simulink library "Feeder3_lib"  (Simulink 8.1)
settings: Solver=ode45  StartTime=0.0  StopTime=10.0  RelTol=1e-3
values from neighbouring files (symbols this model uses):
  DER_REL = xlsread('DER_relay.xlsx')    [relay_settings_init.m]
  Ts = 100E-6    (= 0.0001)    [BANSHEE_init.m]    (also in Ghost_init.m)
undefined symbols (not defined in the file or in its folder): CBID, Left, type, V
libraries: cables_lib x12, breaker_lib x12, powerlib x7, transformer_lib x6, Load_lib x6, ssn_lib x3, PHIL_lib x2, rtio_generic_modbus x2, NREL_Diesel_Genset_lib x2, rtlab x2, powerlib_meascontrol x1, Motor_InductionMachine_lib x1
settings Model: Creator=re25624  LastModifiedBy=hptb1

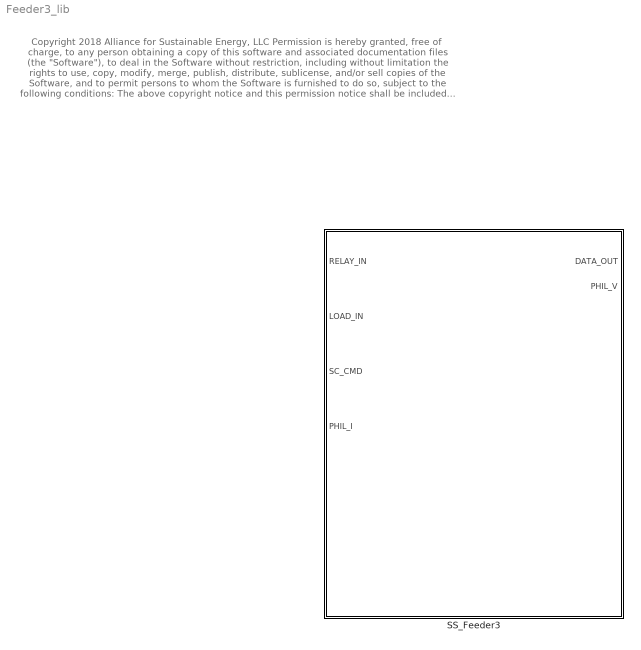
== system Feeder3_lib ==
  note: Copyright 2018 Alliance for Sustainable Energy, LLC
      |
      | Permission is hereby granted, free of charge, to any person obtaining a copy of this software
      | and associated documentation files (the "Software"), to deal in the Software without restriction,
      | including without limitation the rights to use, copy, modify, merge, publish, distribute, sublicense,
      | and/or sell copies of the Software, and to permit persons to whom the Software is furnished to do so,
      | subject to the following conditions:
      |
      | The above copyright notice and this permission notice shall be included in all copies or substantial portions of the Software.
      |
      | THE SOFTWARE IS PROVIDED "AS IS", WITHOUT WARRANTY OF ANY KIND, EXPRESS OR IMPLIED, INCLUDING
      | BUT NOT LIMITED TO THE WARRANTIES OF MERCHANTABILITY, FITNESS FOR A PARTICULAR PURPOSE AND
      | NONINFRINGEMENT. IN NO EVENT SHALL THE AUTHORS, THE COPYRIGHT HOLDERS, THE UNITED STATES,
      | THE UNITED STATES DEPARTMENT OF ENERGY, OR ANY OF THEIR EMPLOYEES BE LIABLE FOR ANY CLAIM,
      | DAMAGES OR OTHER LIABILITY, WHETHER IN AN ACTION OF CONTRACT, TORT OR OTHERWISE, ARISING FROM,
      | OUT OF OR IN CONNECTION WITH THE SOFTWARE OR THE USE OR OTHER DEALINGS IN THE SOFTWARE.
  SS_Feeder3 : Subsystem

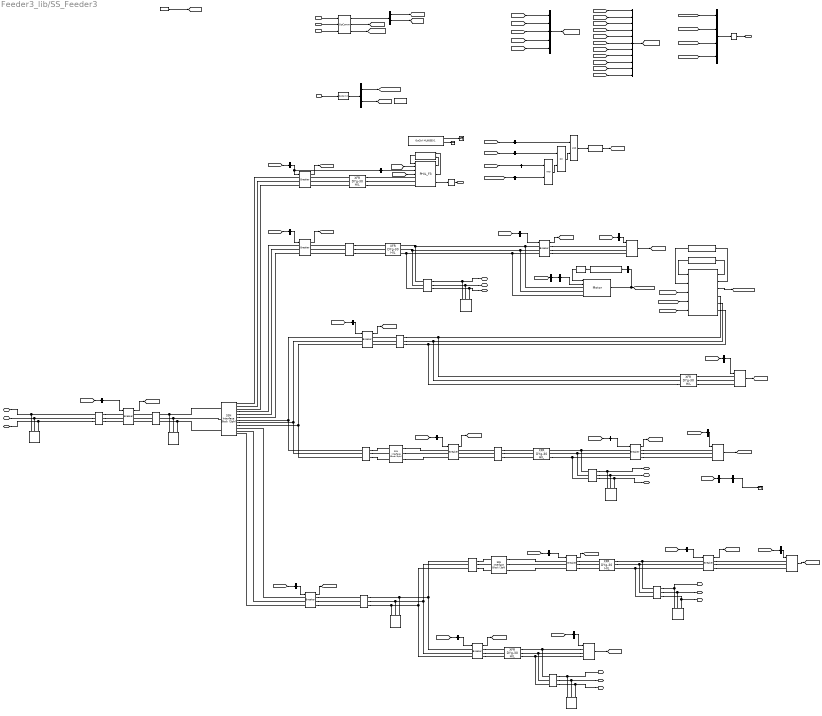
== system Feeder3_lib/SS_Feeder3 ==
  note: Copyright 2018 Alliance for Sustainable Energy, LLC
      |
      | Permission is hereby granted, free of charge, to any person obtaining a copy of this software
      | and associated documentation files (the "Software"), to deal in the Software without restriction,
      | including without limitation the rights to use, copy, modify, merge, publish, distribute, sublicense,
      | and/or sell copies of the Software, and to permit persons to whom the Software is furnished to do so,
      | subject to the following conditions:
      |
      | The above copyright notice and this permission notice shall be included in all copies or substantial portions of the Software.
      |
      | THE SOFTWARE IS PROVIDED "AS IS", WITHOUT WARRANTY OF ANY KIND, EXPRESS OR IMPLIED, INCLUDING
      | BUT NOT LIMITED TO THE WARRANTIES OF MERCHANTABILITY, FITNESS FOR A PARTICULAR PURPOSE AND
      | NONINFRINGEMENT. IN NO EVENT SHALL THE AUTHORS, THE COPYRIGHT HOLDERS, THE UNITED STATES,
      | THE UNITED STATES DEPARTMENT OF ENERGY, OR ANY OF THEIR EMPLOYEES BE LIABLE FOR ANY CLAIM,
      | DAMAGES OR OTHER LIABILITY, WHETHER IN AN ACTION OF CONTRACT, TORT OR OTHERWISE, ARISING FROM,
      | OUT OF OR IN CONNECTION WITH THE SOFTWARE OR THE USE OR OTHER DEALINGS IN THE SOFTWARE.
  note: PHIL interface
  note: connect to F1
  note: connect to F2
  note: connect to F2
  note: connect to F2
  note: Signal for this Cb will come from a SEL relay
  note: Logic to protect against situation where there is no voltage
      | source at F3 side of PHIL. If no voltage source is available current is not injected back to F3
  RELAY_IN : Inport
  LOAD_IN : Inport  Port=2
  SC_CMD : Inport  Port=3
  PHIL_I : Inport  Port=4
  1000 kVA : transformer_lib/XFR DYg-30 HIL  Rating=1000  Vp=13800  Vs=480  Z=5.56  XR=5.49
  1000 kVA1 : transformer_lib/XFR DYg-30 HIL  Rating=1000  Vp=13800  Vs=480  Z=5.56  XR=5.49
  200 HP chiller compressor : Load_lib/200 HP chiller compressor
  2000 kVA : transformer_lib/XFR DYg-30 HIL  Rating=2000  Vp=13800  Vs=480  Z=5.75  XR=5.7
  2000 kVA1 : transformer_lib/XFR DYg-30 HIL  Rating=2000  Vp=13800  Vs=480  Z=5.75  XR=5.7
  2500 kVA : transformer_lib/XFR DYg-30 HIL  Rating=2500  Vp=13800  Vs=480  Z=5.75  XR=6.6
  2500 kVA1 : transformer_lib/XFR DYg-30 HIL  Rating=5000  Vp=13800  Vs=4160  Z=5.75  XR=6.6
  448 kvar inductor at 13.8kV  to cancel kvar produced by the stublines1 : powerlib/Elements/Three-Phase Parallel RLC Load  LConnTagsString=A|B|C  Configuration=Y (grounded)  NominalVoltage=13800  NominalFrequency=60  ActivePower=10e3  InductivePower=448e3  CapacitivePower=0  Measurements=None  LoadType=constant Z
  5 kvar inductor at 480V  to cancel kvar produced by the stublines : powerlib/Elements/Three-Phase Parallel RLC Load  LConnTagsString=A|B|C  Configuration=Y (grounded)  NominalVoltage=480  NominalFrequency=60  ActivePower=1e3  InductivePower=5e3  CapacitivePower=0  Measurements=None  LoadType=constant Z
  500kcmil-Mutual{1..2,4,9} (4 alike) : cables_lib/500kcmil-Mutual  length=10  par_sets=1  ratio=3
  500kcmil-Mutual3 : cables_lib/500kcmil-Mutual  length=100  par_sets=1  ratio=3
  500kcmil-Mutual5 : cables_lib/500kcmil-Mutual  length=1000  par_sets=1  ratio=3
  6 kvar inductor at 480V  to cancel kvar produced by the stublines1 : powerlib/Elements/Three-Phase Parallel RLC Load  LConnTagsString=A|B|C  Configuration=Y (grounded)  NominalVoltage=480  NominalFrequency=60  ActivePower=1e3  InductivePower=6e3  CapacitivePower=0  Measurements=None  LoadType=constant Z
  6 kvar inductor at 480V  to cancel kvar produced by the stublines2 : powerlib/Elements/Three-Phase Parallel RLC Load  LConnTagsString=A|B|C  Configuration=Y (grounded)  NominalVoltage=480  NominalFrequency=60  ActivePower=1e3  InductivePower=6e3  CapacitivePower=0  Measurements=None  LoadType=constant Z
  6 kvar inductor at 480V  to cancel kvar produced by the stublines3 : powerlib/Elements/Three-Phase Parallel RLC Load  LConnTagsString=A|B|C  Configuration=Y (grounded)  NominalVoltage=480  NominalFrequency=60  ActivePower=0  InductivePower=6e3  CapacitivePower=0  Measurements=None  LoadType=constant Z
  AIN_AOUT_ML605EX1 : PHIL_lib/AIN_AOUT_ML605EX1
  Bus Creator2 : BusCreator
  Bus Creator3 : BusCreator  Inputs=5
  Bus Creator5 : BusCreator  Inputs=11
  Bus Selector : BusSelector  OutputSignals=motor
  Bus Selector1 : BusSelector  OutputSignals=F3_CB_4
  Bus Selector10 : BusSelector  OutputSignals=F3_CB_5
  Bus Selector11 : BusSelector  OutputSignals=P6
  Bus Selector12 : BusSelector  OutputSignals=F3_CB_9
  Bus Selector13 : BusSelector  OutputSignals=F3_CB_3
  Bus Selector14 : BusSelector  OutputSignals=F3_CB_8
  Bus Selector15 : BusSelector  OutputSignals=CHP_cmds,IO_scaling
  Bus Selector17 : BusSelector  OutputSignals=RPM
  Bus Selector18 : BusSelector  OutputSignals=LoadProfile,TestSeq
  Bus Selector19 : BusSelector  OutputSignals=Logic_trip
  Bus Selector2 : BusSelector  OutputSignals=C6
  Bus Selector20 : BusSelector  OutputSignals=ena2
  Bus Selector21 : BusSelector  OutputSignals=F3_PCC
  Bus Selector22 : BusSelector  OutputSignals=F3_CB_10
  Bus Selector23 : BusSelector  OutputSignals=fault
  Bus Selector24 : BusSelector  OutputSignals=loc4
  Bus Selector25 : BusSelector  OutputSignals=Status
  Bus Selector26 : BusSelector  OutputSignals=Status
  Bus Selector27 : BusSelector  OutputSignals=Status
  Bus Selector28 : BusSelector  OutputSignals=cb.cb_meas.Status
  Bus Selector3 : BusSelector  OutputSignals=P4
  Bus Selector4 : BusSelector  OutputSignals=I6
  Bus Selector5 : BusSelector  OutputSignals=C5
  Bus Selector6 : BusSelector  OutputSignals=F3_CB_2
  Bus Selector7 : BusSelector  OutputSignals=F3_CB_7
  Bus Selector8 : BusSelector  OutputSignals=F3_CB_6
  Bus Selector9 : BusSelector  OutputSignals=F3_CB_1
  C1 : cables_lib/500kcmil-Mutual  length=10  par_sets=1  ratio=3
  C2 : cables_lib/500kcmil-Mutual  length=10  par_sets=1  ratio=3
  C301 : cables_lib/500kcmil-Mutual  length=2500  par_sets=1  ratio=3
  C302 : cables_lib/4//0AWG-Mutual  length=2000  par_sets=1  ratio=3
  C303 : cables_lib/500kcmil-Mutual  length=2000  par_sets=1  ratio=3
  C304 : cables_lib/4//0AWG-Mutual  length=1500  par_sets=2  ratio=3
  CHP_Modbus : rtio_generic_modbus/Modbus device  conf_name=CHP_modbus.opal  conf_name_mask=CHP_modbus.xls  sample_time=Ts
  Critical_5 : Load_lib/Dynamic_Load  V=480  kVA=1000  PF=0.9  Ts=Ts
  Critical_6 : Load_lib/Dynamic_Load  V=480  kVA=800  PF=0.9  Ts=Ts
  Data Type Conversion : DataTypeConversion  OutDataTypeStr=double
  F3_CB_{1..6,8..11} (10 alike) : breaker_lib/Breaker  Ts=Ts  mech_delay=cb_mech_delay
  F3_PCC : breaker_lib/Breaker  Ts=Ts  mech_delay=cb_mech_delay
  First-Order Filter : powerlib_meascontrol/Filters/First-Order Filter  FilterType=Lowpass  Tc=10e-3  Ts=Ts  Initialize=on  Vac_Init=[0, 0, 60]  Vdc_Init=0  PlotResponse=off  FreqRange="[0,  200,  1]"
  GEN2_Modbus : rtio_generic_modbus/Modbus device  conf_name=GEN2_modbus.opal  conf_name_mask=GEN2_modbus.xls  sample_time=Ts
  Goto Tag Visibility : GotoTagVisibility  GotoTag=phil_ctrl
  Interruptible_6 : Load_lib/Dynamic_Load  V=480  kVA=600  PF=0.9  Ts=Ts
  Logical Operator : Logic  AllPortsSameDT=off  OutDataTypeStr=boolean
  Logical Operator1 : Logic  Operator=OR  AllPortsSameDT=off  OutDataTypeStr=boolean
  Logical Operator2 : Logic  AllPortsSameDT=off  OutDataTypeStr=boolean
  Losses1 : powerlib/Elements/Three-Phase Parallel RLC Load  LConnTagsString=A|B|C  Configuration=Y (grounded)  NominalVoltage=13800  NominalFrequency=60  ActivePower=1e3  InductivePower=0  CapacitivePower=0  Measurements=None  LoadType=constant Z
  Losses4 : powerlib/Elements/Three-Phase Parallel RLC Load  LConnTagsString=A|B|C  Configuration=Y (grounded)  NominalVoltage=13800  NominalFrequency=60  ActivePower=1e3  InductivePower=0  CapacitivePower=0  Measurements=None  LoadType=constant Z
  Memory : Memory
  Memory1 : Memory
  Motor : Motor_InductionMachine_lib/Motor
  NGCHP_Generator : Subsystem
  OpComm1 : rtlab/OpComm  nbport=3  groupe_acq=1  subsys_rate=0  st=0  Synchronization=on  Interpolation=on  Threshold=1.0  Missed_Data=off  Sim_Time=off  Samples=off  dynSigOut=off  from_console=0  warning_done=off  writeOpCommFile=off  Offset=off
  OpComm2 : rtlab/OpComm  nbport=1  groupe_acq=1  subsys_rate=0  st=0  Synchronization=on  Interpolation=on  Threshold=1.0  Missed_Data=off  Sim_Time=off  Samples=off  dynSigOut=off  from_console=1  warning_done=off  writeOpCommFile=off  Offset=off
  OpCtrl ML605EX1 : rtio_opalrt_ml605ex1/OpCtrl ML605EX1  CtrlName='ML605EX1 Ctrl'  boardid=4  BitstreamFilename=ML605_2-EX-0029-2_2_4_33-32AIO_16DIO16SelectableDIO-10-01.bin  numconfig=-1  mode=Master  externalClock=off  decimRtsi=0  calibIO=off  SampleTime=0  loadinport=-1
  PHIL_F3 : PHIL_lib/PHIL_F3
  Priority_4 : Load_lib/Dynamic_Load  V=480  kVA=600  PF=0.9  Ts=Ts
  Priority_6 : Load_lib/Dynamic_Load  V=480  kVA=1000  PF=0.9  Ts=Ts
  SSN Interface Block (3ph)1 : ssn_lib/SSN Interface Block (3ph)  nb_phase=3  nb_port=2  p1_type=V-type(Left)  p2_type=V-type (Right)  p3_type=V-type(Left)  p4_type=V-type(Left)  p5_type=V-type(Left)  p6_type=V-type(Left)  p7_type=V-type(Left)  p8_type=V-type(Left)  p9_type=V-type(Left)  p10_type=V-type(Left)  p11_type=V-type(Left)  p12_type=V-type(Left)  p13_type=V-type(Left)  p14_type=V-type(Left)  p15_type=V-type(Left)  p16_type=V-type(Left)  I_port_shunt_resistance=1e9
  SSN Interface Block (3ph)2 : ssn_lib/SSN Interface Block (3ph)  nb_phase=3  nb_port=2  p1_type=V-type(Left)  p2_type=V-type (Right)  p3_type=V-type(Left)  p4_type=V-type(Left)  p5_type=V-type(Left)  p6_type=V-type(Left)  p7_type=V-type(Left)  p8_type=V-type(Left)  p9_type=V-type(Left)  p10_type=V-type(Left)  p11_type=V-type(Left)  p12_type=V-type(Left)  p13_type=V-type(Left)  p14_type=V-type(Left)  p15_type=V-type(Left)  p16_type=V-type(Left)  I_port_shunt_resistance=1e9
  SSN Interface Block (3ph)5 : ssn_lib/SSN Interface Block (3ph)  nb_phase=3  nb_port=5  p1_type=V-type(Left)  p2_type=V-type (Right)  p3_type=V-type (Right)  p4_type=V-type (Right)  p5_type=V-type (Right)  p6_type=V-type(Left)  p7_type=V-type(Left)  p8_type=V-type(Left)  p9_type=V-type(Left)  p10_type=V-type(Left)  p11_type=V-type(Left)  p12_type=V-type(Left)  p13_type=V-type(Left)  p14_type=V-type(Left)  p15_type=V-type(Left)  p16_type=V-type(Left)  I_port_shunt_resistance=1e9
  "State " : Constant  Value=0
  Terminator : Terminator
  Terminator1 : Terminator
  Terminator5 : Terminator
  A_CB_4 : PMIOPort  Port=1  Side=Right
  B_CB_4 : PMIOPort  Port=2  Side=Right
  C_CB_4 : PMIOPort  Port=3  Side=Right
  A_CB_5 : PMIOPort  Port=4  Side=Right
  B_CB_5 : PMIOPort  Port=5  Side=Right
  C_CB_5 : PMIOPort  Port=6  Side=Right
  A_CB_6 : PMIOPort  Port=7  Side=Right
  B_CB_6 : PMIOPort  Port=8  Side=Right
  C_CB_6 : PMIOPort  Port=9  Side=Right
  A_CB_7 : PMIOPort  Port=10  Side=Right
  B_CB_7 : PMIOPort  Port=11  Side=Right
  C_CB_7 : PMIOPort  Port=12  Side=Right
  PCC_A : PMIOPort  Port=13  Side=Left
  PCC_B : PMIOPort  Port=14  Side=Left
  PCC_C : PMIOPort  Port=15  Side=Left
  DATA_OUT : Outport
  PHIL_V : Outport  Port=2
  tag scope: phil_ctrl=scoped
  wires:
  PHIL_F3/2 -> AIN_AOUT_ML605EX1/1
  Data Type Conversion/1 -> [Vsrc_con]
  [Vsrc_con] -> PHIL_F3/4
  Logical Operator/1 -> Data Type Conversion/1
  Logical Operator1/1 -> Logical Operator/2
  Logical Operator2/1 -> Logical Operator1/2
  Bus Selector27/1 -> Logical Operator2/1  "<Status>"
  Bus Selector28/1 -> Logical Operator2/2  "<Status>"
  [NG_CHP_DATA] -> Bus Selector28/1
  Bus Selector26/1 -> Logical Operator1/1  "<Status>"
  [F3_PCC] -> Bus Selector26/1
  Bus Selector25/1 -> Logical Operator/1  "<Status>"
  [F3_CB_3] -> Bus Selector27/1  "F3_CB_3"
  [F3_CB_10] -> Bus Selector25/1
  Bus Selector24/1 -> Terminator5/1  "<loc4>"
  Bus Selector23/1 -> Bus Selector24/1  "<fault>"
  [TestSeq] -> Bus Selector23/1
  AIN_AOUT_ML605EX1/1 -> PHIL_F3/1
  PHIL_F3/1 -> AIN_AOUT_ML605EX1/2
  First-Order Filter/1 -> Motor/1
  [TestSeq] -> NGCHP_Generator/5(testseq)
  [MOTOR_DATA] -> Bus Creator2/4  "MOTOR_DATA"
  Motor/1 -> [MOTOR_DATA], Bus Selector17/1
  OpCtrl ML605EX1/2 -> Terminator1/1
  OpCtrl ML605EX1/1 -> Terminator/1
  Bus Selector15/2 -> [phil_ctrl]  "<IO_scaling>"
  Bus Selector20/1 -> Motor/2  "<ena2>"
  [PHIL_I] -> PHIL_F3/2
  Bus Selector19/1 -> PHIL_F3/3  "<Logic_trip>"
  PHIL_F3/3 -> Memory1/1
  Memory1/1 -> PHIL_V/1
  Bus Selector22/1 -> F3_CB_10/1, Bus Selector19/1  "<F3_CB_10>"
  F3_CB_10/1 -> [F3_CB_10]
  Bus Selector18/2 -> [TestSeq]  "<TestSeq>"
  Bus Selector18/1 -> [LOAD_IN]  "<LoadProfile>"
  PHIL_I/1 -> OpComm1/3
  OpComm1/3 -> [PHIL_I]
  [F3_CB_10] -> Bus Creator5/10  "F3_CB_10"
  [RELAY_IN] -> Bus Selector22/1
  Bus Selector15/1 -> [NGCHP_Gen]  "<CHP_cmds>"
  CHP_Modbus/1 -> NGCHP_Generator/2(ModbusIn1)
  NGCHP_Generator/2(ModbusOutCHP) -> CHP_Modbus/1
  [heat_load] -> NGCHP_Generator/4(Heat Load MBtu/hrs)
  NGCHP_Generator/3(Gen_meas) -> [NG_CHP_DATA]
  NGCHP_Generator/1(ModbusOut) -> GEN2_Modbus/1  "Gen_meas"
  GEN2_Modbus/1 -> NGCHP_Generator/1(ModbusIn)
  [NGCHP_Gen] -> NGCHP_Generator/3(console)
  [RELAY_IN] -> Bus Selector21/1
  Bus Selector21/1 -> F3_PCC/1  "<F3_PCC>"
  Bus Selector/1 -> Bus Selector20/1  "<motor>"
  [TestSeq] -> Bus Selector/1
  200 HP chiller compressor/1 -> First-Order Filter/1
  Bus Selector17/1 -> 200 HP chiller compressor/1  "<RPM>"
  [NG_CHP_DATA] -> Bus Creator2/3  "NG_CHP_DATA"
  [LOAD_DATA] -> Bus Creator2/2  "LOAD_DATA"
  [CB_DATA] -> Bus Creator2/1  "CB_DATA"
  Bus Creator2/1 -> Memory/1
  OpComm2/1 -> Bus Selector15/1
  "State "/1 -> [heat_load]  "Heat Load MBtu/hr"
  Memory/1 -> DATA_OUT/1
  SC_CMD/1 -> OpComm2/1
  [F3_CB_9] -> Bus Creator5/9  "F3_CB_9"
  [F3_CB_8] -> Bus Creator5/8  "F3_CB_8"
  [RELAY_IN] -> Bus Selector14/1
  Bus Selector14/1 -> F3_CB_8/1  "<F3_CB_8>"
  F3_CB_8/1 -> [F3_CB_8]
  [RELAY_IN] -> Bus Selector12/1
  Bus Selector12/1 -> F3_CB_9/1  "<F3_CB_9>"
  F3_CB_9/1 -> [F3_CB_9]
  [LOAD_P6] -> Bus Creator3/5  "F3_P6"
  Priority_6/1 -> [LOAD_P6]
  Bus Selector11/1 -> Priority_6/1  "<P6>"
  [LOAD_IN] -> Bus Selector11/1
  [F3_PCC] -> Bus Creator5/11  "F3_PCC"
  F3_PCC/1 -> [F3_PCC]
  F3_CB_11/1 -> [F3_CB_7]
  [RELAY_IN] -> Bus Selector13/1
  Bus Selector13/1 -> F3_CB_3/1  "<F3_CB_3>"
  [RELAY_IN] -> Bus Selector10/1
  Bus Selector10/1 -> F3_CB_5/1  "<F3_CB_5>"
  [RELAY_IN] -> Bus Selector9/1
  Bus Selector9/1 -> F3_CB_1/1  "<F3_CB_1>"
  [RELAY_IN] -> Bus Selector8/1
  Bus Selector8/1 -> F3_CB_6/1  "<F3_CB_6>"
  [RELAY_IN] -> Bus Selector7/1
  Bus Selector7/1 -> F3_CB_11/1  "<F3_CB_7>"
  [RELAY_IN] -> Bus Selector6/1
  Bus Selector6/1 -> F3_CB_2/1  "<F3_CB_2>"
  OpComm1/2 -> [RELAY_IN]
  RELAY_IN/1 -> OpComm1/2
  [RELAY_IN] -> Bus Selector1/1
  Bus Creator5/1 -> [CB_DATA]
  [F3_CB_4] -> Bus Creator5/4  "F3_CB_4"
  [F3_CB_2] -> Bus Creator5/2  "F3_CB_2"
  [F3_CB_3] -> Bus Creator5/3  "F3_CB_3"
  [F3_CB_6] -> Bus Creator5/6  "F3_CB_6"
  [F3_CB_7] -> Bus Creator5/7  "F3_CB_7"
  [F3_CB_5] -> Bus Creator5/5  "F3_CB_5"
  [F3_CB_1] -> Bus Creator5/1  "F3_CB_1"
  F3_CB_5/1 -> [F3_CB_5]
  F3_CB_1/1 -> [F3_CB_1]
  F3_CB_6/1 -> [F3_CB_6]
  F3_CB_2/1 -> [F3_CB_2]
  F3_CB_3/1 -> [F3_CB_3]
  F3_CB_4/1 -> [F3_CB_4]
  Bus Creator3/1 -> [LOAD_DATA]  "LOAD"
  [LOAD_P4] -> Bus Creator3/4  "F3_P4"
  [LOAD_I6] -> Bus Creator3/3  "F3_I6"
  [LOAD_C5] -> Bus Creator3/1  "F3_C5"
  [LOAD_C6] -> Bus Creator3/2  "F3_C6"
  Critical_5/1 -> [LOAD_C5]
  Interruptible_6/1 -> [LOAD_I6]
  Priority_4/1 -> [LOAD_P4]
  Critical_6/1 -> [LOAD_C6]
  Bus Selector5/1 -> Critical_5/1  "<C5>"
  Bus Selector4/1 -> Interruptible_6/1  "<I6>"
  Bus Selector3/1 -> Priority_4/1  "<P4>"
  Bus Selector2/1 -> Critical_6/1  "<C6>"
  [LOAD_IN] -> Bus Selector5/1
  [LOAD_IN] -> Bus Selector4/1
  [LOAD_IN] -> Bus Selector3/1
  [LOAD_IN] -> Bus Selector2/1
  OpComm1/1 -> Bus Selector18/1
  LOAD_IN/1 -> OpComm1/1
  Bus Selector1/1 -> F3_CB_4/1  "<F3_CB_4>"
  connections:
  F3_CB_11/RConn3 -- Priority_4/LConn3
  F3_CB_11/RConn1 -- Priority_4/LConn1
  2500 kVA1/RConn1 -- PHIL_F3/LConn1
  2500 kVA1/RConn2 -- PHIL_F3/LConn2
  2500 kVA1/RConn3 -- PHIL_F3/LConn3
  2500 kVA1/LConn3 -- F3_CB_10/RConn3
  2500 kVA1/LConn1 -- F3_CB_10/RConn1
  2500 kVA1/LConn2 -- F3_CB_10/RConn2
  F3_CB_10/LConn1 -- SSN Interface Block (3ph)5/RConn1
  F3_CB_10/LConn2 -- SSN Interface Block (3ph)5/RConn2
  F3_CB_10/LConn3 -- SSN Interface Block (3ph)5/RConn3
  F3_CB_1/RConn3 -- C301/LConn3
  F3_CB_1/RConn2 -- C301/LConn2
  F3_CB_1/RConn1 -- C301/LConn1
  SSN Interface Block (3ph)1/RConn3 -- F3_CB_6/LConn3
  SSN Interface Block (3ph)1/RConn2 -- F3_CB_6/LConn2
  SSN Interface Block (3ph)1/RConn1 -- F3_CB_6/LConn1
  F3_CB_1/LConn3 -- SSN Interface Block (3ph)5/RConn12
  F3_CB_1/LConn1 -- SSN Interface Block (3ph)5/RConn10
  F3_CB_1/LConn2 -- SSN Interface Block (3ph)5/RConn11
  C2/RConn3 -- SSN Interface Block (3ph)2/LConn3
  C2/RConn1 -- SSN Interface Block (3ph)2/LConn1
  C2/RConn2 -- SSN Interface Block (3ph)2/LConn2
  SSN Interface Block (3ph)2/RConn1 -- F3_CB_2/LConn1
  SSN Interface Block (3ph)2/RConn2 -- F3_CB_2/LConn2
  SSN Interface Block (3ph)2/RConn3 -- F3_CB_2/LConn3
  500kcmil-Mutual5/LConn3 -- 448 kvar inductor at 13.8kV  to cancel kvar produced by the stublines1/LConn3 -- PCC_C/RConn1
  500kcmil-Mutual5/LConn2 -- 448 kvar inductor at 13.8kV  to cancel kvar produced by the stublines1/LConn2 -- PCC_B/RConn1
  448 kvar inductor at 13.8kV  to cancel kvar produced by the stublines1/LConn1 -- 500kcmil-Mutual5/LConn1 -- PCC_A/RConn1
  Losses4/LConn3 -- SSN Interface Block (3ph)5/LConn3 -- 500kcmil-Mutual3/RConn3
  Losses4/LConn2 -- SSN Interface Block (3ph)5/LConn2 -- 500kcmil-Mutual3/RConn2
  Losses4/LConn1 -- SSN Interface Block (3ph)5/LConn1 -- 500kcmil-Mutual3/RConn1
  C1/RConn1 -- SSN Interface Block (3ph)1/LConn1
  C1/RConn3 -- SSN Interface Block (3ph)1/LConn3
  C1/RConn2 -- SSN Interface Block (3ph)1/LConn2
  F3_CB_11/LConn3 -- 1000 kVA/RConn3 -- 500kcmil-Mutual4/LConn3
  500kcmil-Mutual5/RConn3 -- F3_PCC/LConn3
  500kcmil-Mutual5/RConn2 -- F3_PCC/LConn2
  500kcmil-Mutual5/RConn1 -- F3_PCC/LConn1
  500kcmil-Mutual3/LConn2 -- F3_PCC/RConn2
  500kcmil-Mutual3/LConn1 -- F3_PCC/RConn1
  500kcmil-Mutual3/LConn3 -- F3_PCC/RConn3
  B_CB_4/RConn1 -- 500kcmil-Mutual9/RConn2 -- 5 kvar inductor at 480V  to cancel kvar produced by the stublines/LConn2
  C_CB_4/RConn1 -- 500kcmil-Mutual9/RConn3 -- 5 kvar inductor at 480V  to cancel kvar produced by the stublines/LConn3
  A_CB_4/RConn1 -- 500kcmil-Mutual9/RConn1 -- 5 kvar inductor at 480V  to cancel kvar produced by the stublines/LConn1
  A_CB_7/RConn1 -- 500kcmil-Mutual4/RConn1 -- 6 kvar inductor at 480V  to cancel kvar produced by the stublines1/LConn1
  C_CB_7/RConn1 -- 500kcmil-Mutual4/RConn3 -- 6 kvar inductor at 480V  to cancel kvar produced by the stublines1/LConn3
  B_CB_7/RConn1 -- 500kcmil-Mutual4/RConn2 -- 6 kvar inductor at 480V  to cancel kvar produced by the stublines1/LConn2
  500kcmil-Mutual2/RConn1 -- A_CB_6/RConn1 -- 6 kvar inductor at 480V  to cancel kvar produced by the stublines2/LConn1
  C_CB_6/RConn1 -- 500kcmil-Mutual2/RConn3 -- 6 kvar inductor at 480V  to cancel kvar produced by the stublines2/LConn3
  B_CB_6/RConn1 -- 500kcmil-Mutual2/RConn2 -- 6 kvar inductor at 480V  to cancel kvar produced by the stublines2/LConn2
  C_CB_5/RConn1 -- 500kcmil-Mutual1/RConn3 -- 6 kvar inductor at 480V  to cancel kvar produced by the stublines3/LConn3
  6 kvar inductor at 480V  to cancel kvar produced by the stublines3/LConn1 -- 500kcmil-Mutual1/RConn1 -- A_CB_5/RConn1
  B_CB_5/RConn1 -- 500kcmil-Mutual1/RConn2 -- 6 kvar inductor at 480V  to cancel kvar produced by the stublines3/LConn2
  1000 kVA1/RConn3 -- Critical_6/LConn3
  1000 kVA1/RConn2 -- Critical_6/LConn2
  1000 kVA1/RConn1 -- Critical_6/LConn1
  C303/RConn1 -- 2500 kVA/LConn1
  C303/RConn3 -- 2500 kVA/LConn3
  C303/RConn2 -- 2500 kVA/LConn2
  C303/LConn3 -- F3_CB_4/RConn3
  C303/LConn2 -- F3_CB_4/RConn2
  C303/LConn1 -- F3_CB_4/RConn1
  SSN Interface Block (3ph)5/RConn8 -- F3_CB_3/LConn2 -- C2/LConn2
  SSN Interface Block (3ph)5/RConn9 -- F3_CB_3/LConn3 -- C2/LConn3
  SSN Interface Block (3ph)5/RConn7 -- F3_CB_3/LConn1 -- C2/LConn1
  SSN Interface Block (3ph)5/RConn5 -- F3_CB_4/LConn2
  SSN Interface Block (3ph)5/RConn6 -- F3_CB_4/LConn3
  SSN Interface Block (3ph)5/RConn4 -- F3_CB_4/LConn1
  F3_CB_8/RConn3 -- Interruptible_6/LConn3
  F3_CB_8/RConn2 -- Interruptible_6/LConn2
  F3_CB_8/RConn1 -- Interruptible_6/LConn1
  F3_CB_9/RConn3 -- Priority_6/LConn3
  F3_CB_9/RConn2 -- Priority_6/LConn2
  F3_CB_9/RConn1 -- Priority_6/LConn1
  1000 kVA/RConn1 -- F3_CB_11/LConn1 -- 500kcmil-Mutual4/LConn1
  F3_CB_11/LConn2 -- 1000 kVA/RConn2 -- 500kcmil-Mutual4/LConn2
  C304/RConn1 -- 1000 kVA/LConn1
  C304/RConn3 -- 1000 kVA/LConn3
  C304/RConn2 -- 1000 kVA/LConn2
  F3_CB_9/LConn2 -- 2500 kVA/RConn2 -- 500kcmil-Mutual9/LConn2 -- Motor/LConn2
  2500 kVA/RConn3 -- 500kcmil-Mutual9/LConn3 -- F3_CB_9/LConn3 -- Motor/LConn3
  F3_CB_9/LConn1 -- 2500 kVA/RConn1 -- 500kcmil-Mutual9/LConn1 -- Motor/LConn1
  Critical_5/LConn2 -- 500kcmil-Mutual1/LConn2 -- 2000 kVA/RConn2
  Critical_5/LConn3 -- 500kcmil-Mutual1/LConn3 -- 2000 kVA/RConn3
  Critical_5/LConn1 -- 500kcmil-Mutual1/LConn1 -- 2000 kVA/RConn1
  F3_CB_8/LConn2 -- 500kcmil-Mutual2/LConn2 -- 2000 kVA1/RConn2
  F3_CB_8/LConn3 -- 2000 kVA1/RConn3 -- 500kcmil-Mutual2/LConn3
  F3_CB_8/LConn1 -- 500kcmil-Mutual2/LConn1 -- 2000 kVA1/RConn1
  F3_CB_11/RConn2 -- Priority_4/LConn2
  C304/LConn3 -- F3_CB_2/RConn3
  F3_CB_5/RConn3 -- 2000 kVA/LConn3
  F3_CB_5/RConn1 -- 2000 kVA/LConn1
  C302/LConn1 -- F3_CB_3/RConn1
  F3_CB_6/RConn1 -- 2000 kVA1/LConn1
  C304/LConn2 -- F3_CB_2/RConn2
  Losses1/LConn2 -- C301/RConn2 -- F3_CB_5/LConn2 -- C1/LConn2
  C302/LConn3 -- F3_CB_3/RConn3
  F3_CB_5/RConn2 -- 2000 kVA/LConn2
  NGCHP_Generator/RConn2 -- 1000 kVA1/LConn2 -- C302/RConn2
  F3_CB_6/RConn2 -- 2000 kVA1/LConn2
  NGCHP_Generator/RConn1 -- 1000 kVA1/LConn1 -- C302/RConn1
  C302/LConn2 -- F3_CB_3/RConn2
  1000 kVA1/LConn3 -- NGCHP_Generator/RConn3 -- C302/RConn3
  C304/LConn1 -- F3_CB_2/RConn1
  Losses1/LConn1 -- C301/RConn3 -- F3_CB_5/LConn3 -- C1/LConn3
  F3_CB_6/RConn3 -- 2000 kVA1/LConn3
  Losses1/LConn3 -- C301/RConn1 -- F3_CB_5/LConn1 -- C1/LConn1

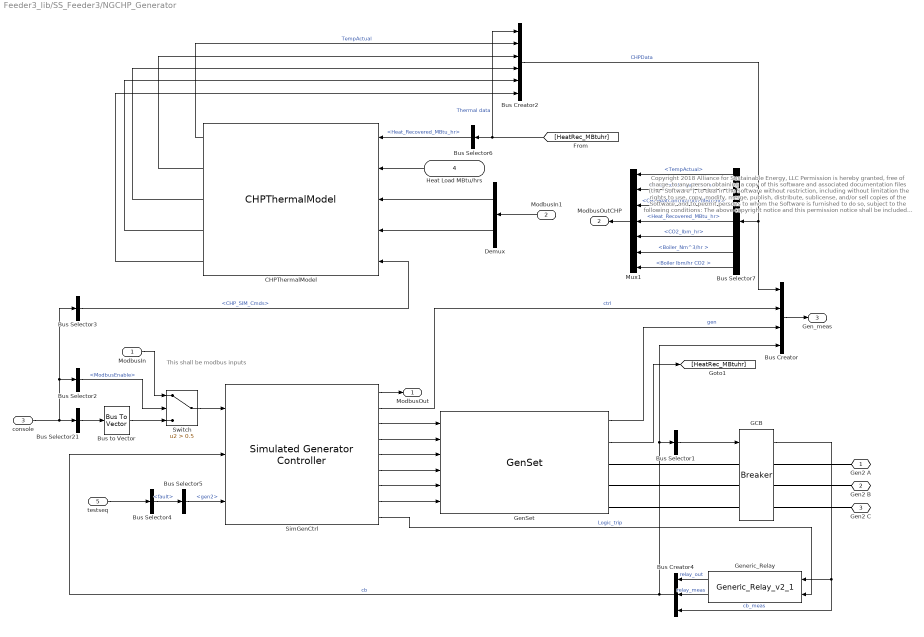
== system Feeder3_lib/SS_Feeder3/NGCHP_Generator ==
  note: Copyright 2018 Alliance for Sustainable Energy, LLC
      |
      | Permission is hereby granted, free of charge, to any person obtaining a copy of this software
      | and associated documentation files (the "Software"), to deal in the Software without restriction,
      | including without limitation the rights to use, copy, modify, merge, publish, distribute, sublicense,
      | and/or sell copies of the Software, and to permit persons to whom the Software is furnished to do so,
      | subject to the following conditions:
      |
      | The above copyright notice and this permission notice shall be included in all copies or substantial portions of the Software.
      |
      | THE SOFTWARE IS PROVIDED "AS IS", WITHOUT WARRANTY OF ANY KIND, EXPRESS OR IMPLIED, INCLUDING
      | BUT NOT LIMITED TO THE WARRANTIES OF MERCHANTABILITY, FITNESS FOR A PARTICULAR PURPOSE AND
      | NONINFRINGEMENT. IN NO EVENT SHALL THE AUTHORS, THE COPYRIGHT HOLDERS, THE UNITED STATES,
      | THE UNITED STATES DEPARTMENT OF ENERGY, OR ANY OF THEIR EMPLOYEES BE LIABLE FOR ANY CLAIM,
      | DAMAGES OR OTHER LIABILITY, WHETHER IN AN ACTION OF CONTRACT, TORT OR OTHERWISE, ARISING FROM,
      | OUT OF OR IN CONNECTION WITH THE SOFTWARE OR THE USE OR OTHER DEALINGS IN THE SOFTWARE.
  note: This shall be modbus inputs
  ModbusIn : Inport
  ModbusIn1 : Inport  Port=2
  console : Inport  Port=3
  Heat Load MBtu/hrs : Inport  Port=4
  testseq : Inport  Port=5
  Bus Creator : BusCreator
  Bus Creator2 : BusCreator  Inputs=6
  Bus Creator4 : BusCreator  Inputs=3
  Bus Selector1 : BusSelector  OutputSignals=relay_out  OutputAsBus=on
  Bus Selector2 : BusSelector  OutputSignals=ModbusEnable
  Bus Selector21 : BusSelector  OutputSignals=ModbusFromSC.Ctrl,ModbusFromSC.PCmd,ModbusFromSC.QCmd,ModbusFromSC.VoltCmd,ModbusFromSC.FreqCmd,ModbusFromSC.signal6,ModbusFromSC.signal7,ModbusFromSC.signal8  OutputAsBus=on
  Bus Selector3 : BusSelector  OutputSignals=CHP_SIM_Cmds
  Bus Selector4 : BusSelector  OutputSignals=fault
  Bus Selector5 : BusSelector  OutputSignals=gen2
  Bus Selector6 : BusSelector  OutputSignals=Heat_Recovered_MBtu_hr
  Bus Selector7 : BusSelector  OutputSignals=TempActual,HeatFromBoiler MBtu/hr,CHPHeatContribution MBtu/hr,Thermal data.Heat_Recovered_MBtu_hr,Thermal data.CO2_lbm_hr,Boiler_Nm^3/hr ,Boiler lbm/hr CO2
  Bus to Vector : BusToVector
  CHPThermalModel : CHP_Model_lib/CHPThermalModel  SIM_HIL=SIM_HIL
  Demux : Demux  Outputs=2
  GCB : breaker_lib/Breaker  Ts=Ts  mech_delay=cb_mech_delay
  GenSet : NREL_Diesel_Genset_lib/GenSet  GenSel=3.5MVA natural gas generator
  Generic_Relay : relay_modbus_lib/Generic_Relay_v2_1  Ts=Ts  relay_settings=[DER_REL(CBID.GEN2,:)]
  Mux1 : Mux  Inputs=7
  SimGenCtrl : NREL_Diesel_Genset_lib/Simulated Generator Controller  GenSel=3.5MVA natural gas generator
  Switch : Switch  Criteria=u2 > Threshold  Threshold=0.5
  Gen2 A : PMIOPort  Port=1  Side=Right
  Gen2 B : PMIOPort  Port=2  Side=Right
  Gen2 C : PMIOPort  Port=3  Side=Right
  ModbusOut : Outport
  ModbusOutCHP : Outport  Port=2
  Gen_meas : Outport  Port=3
  wires:
  Bus Selector1/1 -> GCB/1
  Bus Selector5/1 -> SimGenCtrl/3  "<gen2>"
  Bus Selector4/1 -> Bus Selector5/1  "<fault>"
  testseq/1 -> Bus Selector4/1
  Bus Selector3/1 -> CHPThermalModel/5  "<CHP_SIM_Cmds>"
  Bus Creator2/1 -> Bus Selector7/1, Bus Creator/1  "CHPData"
  Bus Selector6/1 -> CHPThermalModel/1  "<Heat_Recovered_MBtu_hr>"
  ModbusIn1/1 -> Demux/1
  [HeatRec_MBtuhr] -> Bus Selector6/1, Bus Creator2/1  "Thermal data"
  CHPThermalModel/3 -> Bus Creator2/4
  Demux/1 -> CHPThermalModel/3
  Mux1/1 -> ModbusOutCHP/1
  Heat Load MBtu/hrs/1 -> CHPThermalModel/2
  Bus Selector7/1 -> Mux1/1  "<TempActual>"
  Bus Selector7/4 -> Mux1/4  "<Heat_Recovered_MBtu_hr>"
  Bus Selector7/5 -> Mux1/5  "<CO2_lbm_hr>"
  Bus Selector7/2 -> Mux1/2  "<HeatFromBoiler MBtu/hr>"
  CHPThermalModel/2 -> Bus Creator2/3
  Demux/2 -> CHPThermalModel/4
  CHPThermalModel/1 -> Bus Creator2/2  "TempActual"
  Bus Selector7/3 -> Mux1/3  "<CHPHeatContribution MBtu/hr>"
  CHPThermalModel/4 -> Bus Creator2/5
  CHPThermalModel/5 -> Bus Creator2/6
  Bus Selector7/7 -> Mux1/7  "<Boiler lbm/hr CO2 >"
  Bus Selector7/6 -> Mux1/6  "<Boiler_Nm^3/hr >"
  GenSet/2 -> [HeatRec_MBtuhr]
  SimGenCtrl/2 -> Bus Creator/2  "ctrl"
  Bus Creator/1 -> Gen_meas/1
  Generic_Relay/2 -> Bus Creator4/2  "relay_meas"
  Generic_Relay/1 -> Bus Creator4/1  "relay_out"
  GCB/1 -> Bus Creator4/3, Generic_Relay/1  "cb_meas"
  Switch/1 -> SimGenCtrl/1
  Bus to Vector/1 -> Switch/3
  Bus Selector21/1 -> Bus to Vector/1
  ModbusIn/1 -> Switch/1
  Bus Selector2/1 -> Switch/2  "<ModbusEnable>"
  console/1 -> Bus Selector3/1, Bus Selector2/1, Bus Selector21/1
  Bus Creator4/1 -> SimGenCtrl/2, Bus Selector1/1, Bus Creator/4  "cb"
  GenSet/1 -> Bus Creator/3  "gen"
  SimGenCtrl/6 -> GenSet/4
  SimGenCtrl/5 -> GenSet/3
  SimGenCtrl/4 -> GenSet/2
  SimGenCtrl/3 -> GenSet/1
  SimGenCtrl/7 -> GenSet/5
  SimGenCtrl/8 -> GenSet/6
  SimGenCtrl/1 -> ModbusOut/1
  SimGenCtrl/9 -> Generic_Relay/2  "Logic_trip"
  connections:
  GenSet/RConn3 -- GCB/LConn3
  GenSet/RConn2 -- GCB/LConn2
  GenSet/RConn1 -- GCB/LConn1
  Gen2 C/RConn1 -- GCB/RConn3
  GCB/RConn2 -- Gen2 B/RConn1
  Gen2 A/RConn1 -- GCB/RConn1
